simulink model "ES300A_SinVltgGenn"  (R2013b)
settings: Solver=FixedStepDiscrete  StartTime=0.0  StopTime=5  RelTol=1e-3
values from neighbouring files (symbols this model uses):
  ELECGLBPRM_PWMPERDMAX_NANOSEC_U32 = DataDict.ConfigParam    [ES300A_SinVltgGenn_DataDict.m]
  ELECGLBPRM_PWMPERDMIN_NANOSEC_U32 = DataDict.ConfigParam    [ES300A_SinVltgGenn_DataDict.m]
  SINVLTGGENN120DEG_MOTREVELEC_F32 = DataDict.Constant    [ES300A_SinVltgGenn_DataDict.m]
  SINVLTGGENN240DEG_MOTREVELEC_F32 = DataDict.Constant    [ES300A_SinVltgGenn_DataDict.m]
  SINVLTGGENN60DEG_MOTREVELEC_F32 = DataDict.Constant    [ES300A_SinVltgGenn_DataDict.m]
  SINVLTGGENNCMUOFFSTBLX_ULS_F32 = DataDict.Constant    [ES300A_SinVltgGenn_DataDict.m]
  SINVLTGGENNCMUOFFSTBLY_NANOSEC_F32 = DataDict.Constant    [ES300A_SinVltgGenn_DataDict.m]
  SinVltgGennDthrLpFilCoeff = DataDict.Calibration    [ES300A_SinVltgGenn_DataDict.m]
  SINVLTGGENNPHAONTIMAXLIM_NANOSEC_U32 = DataDict.Constant    [ES300A_SinVltgGenn_DataDict.m]
  SINVLTGGENNPHAONTISUMMAXLIM_NANOSEC_U32 = DataDict.Constant    [ES300A_SinVltgGenn_DataDict.m]
  SINVLTGGENNPHATOGNDTBL_CNT_U16 = DataDict.Constant    [ES300A_SinVltgGenn_DataDict.m]
  SINVLTGGENNPHATOGNDTBLSIZE_CNT_U16 = DataDict.Constant    [ES300A_SinVltgGenn_DataDict.m]
  SINVLTGGENNSEEDINI_ULS_F32 = DataDict.Constant    [ES300A_SinVltgGenn_DataDict.m]
  SINVLTGGENNSEEDMPLR_ULS_U08 = DataDict.Constant    [ES300A_SinVltgGenn_DataDict.m]
  SINVLTGGENNSEEDOFFS_ULS_F32 = DataDict.Constant    [ES300A_SinVltgGenn_DataDict.m]
  SINVLTGGENNZERODEG_MOTREVELEC_F32 = DataDict.Constant    [ES300A_SinVltgGenn_DataDict.m]
libraries: simulink x10, FixdToFloat x2
(part 1 of 2)
Description:
  | The High Load Stall Thermal Management algorithm protects the system from prolonged intervals of high
  | assist torque at near-stall conditions. In other words, it quickly limits large torque commands if the motor
  | velocity is below a calibratable threshold.
  |      The algorithm uses a low-pass filter (LPF) and a torque limit table to reduce the maximum allowed torque
  | command under certain operating conditions. When motor velocity is equal to or falls below the calibratable
  | threshold, the torque command is applied to the input of the low-pass filter. The output of the filter ramps up
  | and indexes into the torque limit table. The output of this table is the maximum allowed torque command. A
  | slew limit calibration governs the transition rate of the table output.
settings Model: Creator=Prerit Pramod  LastModifiedBy=wzvp6q
settings Model: ModifiedHistory=|
  | 001
  | Initial Release in new model form and new FDD structures for EA 3.0.
  | J. Kleinau
  | 13-Jun-2011
  | n/a
  | 
  | 001B
  | Revised name of input signal from PreLimitTorque to PreLimitforStall to match outputs of SF-04 Assist Sum & Limiting. Updated all references in text and on figures.
  | J. Kleinau
  | 02-Sep-2011
  | n/a
  | 
  | 002
  | Added input for serial communation service to defeat function plus definition. Cleaned up inconsistent names between sections on outputs between sections and made sure wording matched new figure names. Added Serial Comm Defeat Sub-Function section 5.5.
  | J. Kleinau
  | 08-Sep-2011
  | n/a
  | (Systems Approval and Date (N/A if not an SF FDD): Julie A. Kleinau, 08-Sep-2011; Final Approval and Date: M. Kushion, 26-Sep-2011, v002)
  | 
  | 003
  | Converted the function to a model based FDD.
  | P. Pramod
  | 09-Apr-2013
  | ICR-4051
settings DataIOCC: LimitDataPoints=off  SignalLoggingSaveFormat=ModelDataLogs  DSMLogging=off
settings OptimizationCC: ExpressionDepthLimit=2147483647
settings DebuggingCC: FcnCallInpInsideContextMsg=UseLocalSettings  StateNameClashWarn=warning
settings GRTTargetCC: CombineOutputUpdateFcns=off  GRTInterface=on

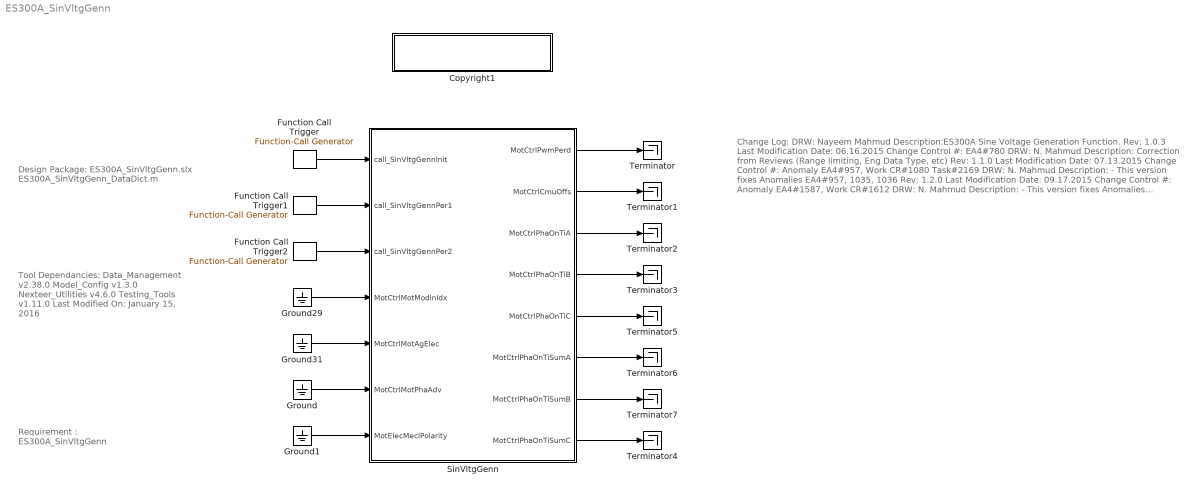
== system ES300A_SinVltgGenn ==
  note: Design Package:
      |
      | ES300A_SinVltgGenn.slx
      | ES300A_SinVltgGenn_DataDict.m
  note: Tool Dependancies:
      |
      | Data_Management v2.38.0
      | Model_Config v1.3.0
      | Nexteer_Utilities v4.6.0
      | Testing_Tools v1.11.0
      |
      | Last Modified On:
      | January 15, 2016
  note: Requirement :
      |
      | ES300A_SinVltgGenn
  note: Change Log:
      |
      | DRW: Nayeem Mahmud
      | Description:ES300A Sine Voltage Generation Function.
      |
      | Rev: 1.0.3
      | Last Modification Date: 06.16.2015
      | Change Control #: EA4#780
      | DRW: N. Mahmud
      | Description: Correction from Reviews (Range limiting, Eng Data Type, etc)
      |
      | Rev: 1.1.0
      | Last Modification Date: 07.13.2015
      | Change Control #: Anomaly EA4#957, Work CR#1080 Task#2169
      | DRW: N. Mahmud
      | Description:
      | - This version fixes  Anomalies EA4#957, 1035, 1036
      |
      | Rev: 1.2.0
      | Last Modification Date: 09.17.2015
      | Change Control #: Anomaly EA4#1587, Work CR#1612
      | DRW: N. Mahmud
      | Description:
      | - This version fixes  Anomalies EA4#1587 by removing the scaling factors for Qax, Dax
      |
      | Rev: 1.3.0
      | Last Modification Date: 01.15.2016
      | Change Control #: Anomaly EA4#1966, Work CR# EA4#3326
      | DRW: N. Mahmud
      | Description:
      | - This version fixes Anomaly EA4#1966 and clarified the requirement to
      | generate Phase On Time for the MIL testing purpose and re-establing the requirement linkage.
      | - Minor Fix: MotCtrlMotAgCorrd has been replaced by MotCtrlMotAgElec in the FR docuemnt
      |
      |
      | Rev: 1.4.0
      | Last Modification Date: 03.11.2016
      | Change Control #: Anomaly EA4#3947, Work CR# EA4#4470
      | DRW: N. Mahmud
      | Description:
      | - This version fixes Anomaly EA4#3947 for low path coverage iussue - the range of
      |  the PhaDptOffsX has been changed to -0.9999847412 to +0.9999847412 in the m-file
      |
      | Rev: 1.5.0
      | Last Modification Date: 05.06.2016
      | Change Control #: Anomaly EA4#4302, Work CR# EA4#5697
      | DRW: G.McCann
      | Description:
      | - This version fixes Anomaly EA4#4302 for .m file TestTolerance = 0 on various output signals.
      | Change to TestTolerance = 1
      | - Add datatype conversion for MotCtrlMotAgElec and MotCtrlMotPhaAdv in SinVltgGennPer1
  Copyright1 : Subsystem  Description=|  mask(Copyright Information){none=on}
      | Copyright info block.                                               
      |                                                                     
      | Place copyright information at the top of every subsystem in design.
      mask prompts: none "No parameters"
      mask help: Place copyright information at the top of every subsystem in design.
      mask Display:
      | NxtrConf = 'Nexteer Confidential';
      | 
      | sys = bdroot; %handle for the current model ("system")
      | first = get_param(sys,'Created');
      | if(isempty(first))
      |     first = datestr(now,'yyyy');
      | else
      |     first = first(end-3:end);  %year is last four digits
      | end
      | 
      | last = get_param(sys,'LastModifiedDate');
      | if isempty(last)
      |     last = datestr(now,'yyyy');
      | else
      |     last = last(end-3:end);
      | end
      | 
      | if strcmp(first,last)
      |     fprintf('%s\nCopyright  %s Nexteer',NxtrConf,first);
      | else
      |     fprintf('%s\n%s%s-%s Nexteer',NxtrConf,char(169),first,last);
      | end
  Function Call Trigger : simulink/Ports & Subsystems/Function-Call Generator  RequirementInfo={} %GIDa_42b49f65_b7bc_4fe6_8fce_d35bfefa497c  sample_time=0.000125  numberOfIterations=1
  Function Call Trigger1 : simulink/Ports & Subsystems/Function-Call Generator  RequirementInfo={} %GIDa_eccf4da5_56c7_476c_afa9_48737326cc68  sample_time=.0000625  numberOfIterations=1
  Function Call Trigger2 : simulink/Ports & Subsystems/Function-Call Generator  RequirementInfo={} %GIDa_73db9335_95f9_41b5_8685_380b234a43a2  sample_time=.0000625  numberOfIterations=1
  Ground{,1,29,31} (4 alike) : Ground
  SinVltgGenn : Subsystem
  Terminator{,1..7} (8 alike) : Terminator
  wires:
  SinVltgGenn/1(MotCtrlPwmPerd) -> Terminator/1
  SinVltgGenn/2(MotCtrlCmuOffs) -> Terminator1/1
  SinVltgGenn/3(MotCtrlPhaOnTiA) -> Terminator2/1
  SinVltgGenn/4(MotCtrlPhaOnTiB) -> Terminator3/1
  SinVltgGenn/5(MotCtrlPhaOnTiC) -> Terminator5/1
  SinVltgGenn/6(MotCtrlPhaOnTiSumA) -> Terminator6/1
  SinVltgGenn/7(MotCtrlPhaOnTiSumB) -> Terminator7/1
  SinVltgGenn/8(MotCtrlPhaOnTiSumC) -> Terminator4/1
  Function Call Trigger/1 -> SinVltgGenn/1(call_SinVltgGennInit)
  Ground1/1 -> SinVltgGenn/7(MotElecMeclPolarity)
  Ground31/1 -> SinVltgGenn/5(MotCtrlMotAgElec)
  Ground/1 -> SinVltgGenn/6(MotCtrlMotPhaAdv)
  Function Call Trigger1/1 -> SinVltgGenn/2(call_SinVltgGennPer1)
  Ground29/1 -> SinVltgGenn/4(MotCtrlMotModlnIdx)
  Function Call Trigger2/1 -> SinVltgGenn/3(call_SinVltgGennPer2)

== system ES300A_SinVltgGenn/Copyright1 ==

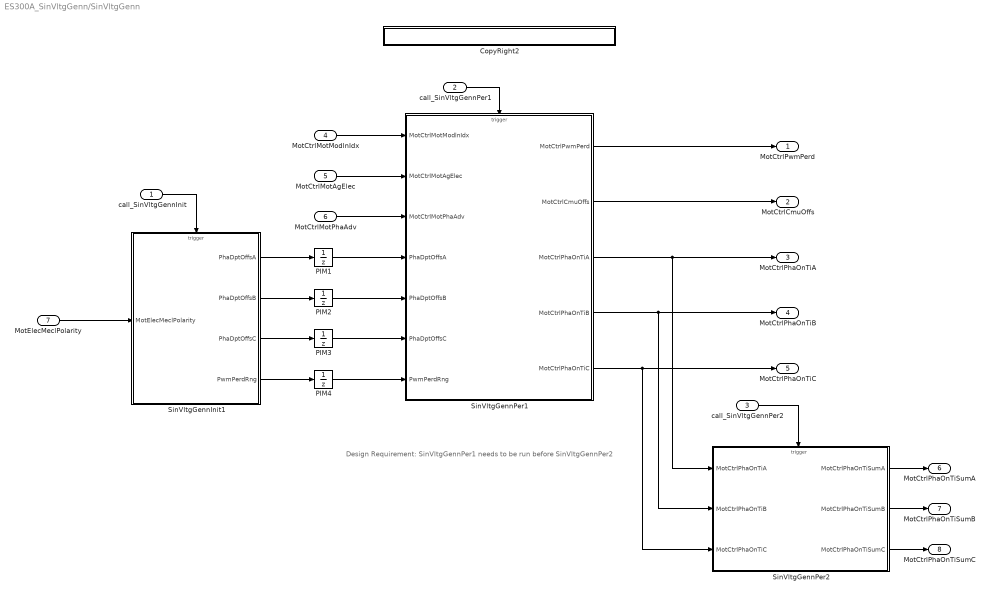
== system ES300A_SinVltgGenn/SinVltgGenn ==
  note: Design Requirement:
      |
      | SinVltgGennPer1 needs to be run before SinVltgGennPer2
  call_SinVltgGennInit : Inport
  call_SinVltgGennPer1 : Inport  RequirementInfo={'linktype_rmi_doors' '0000c478 (/ESG Group/FDD Module Requirements/EA4 Specific/ES300A_SinVltgGenn)' '#ES300A_262' 'true' 'REQ: ES300A_262' '' } %GIDa_f246c4bc_b01d_46bd_87fd_7bc120c20cb6  Port=2
  call_SinVltgGennPer2 : Inport  RequirementInfo={'linktype_rmi_doors' '0000c478 (/ESG Group/FDD Module Requirements/EA4 Specific/ES300A_SinVltgGenn)' '#ES300A_262' 'true' 'REQ: ES300A_262' '' } %GIDa_cb07c873_dffe_45e9_bd8a_092986eec373  Port=3
  MotCtrlMotModlnIdx : Inport  RequirementInfo={'linktype_rmi_doors' '0000c478 (/ESG Group/FDD Module Requirements/EA4 Specific/ES300A_SinVltgGenn)' '#ES300A_104' 'true' 'REQ: ES300A_104' '' } %GIDa_ad60892a_cd90_4ca1_a013_796fa50b9f6b  Port=4
  MotCtrlMotAgElec : Inport  RequirementInfo={'linktype_rmi_doors' '0000c478 (/ESG Group/FDD Module Requirements/EA4 Specific/ES300A_SinVltgGenn)' '#ES300A_103' 'true' 'REQ: ES300A_103' '' } %GIDa_4b3e113f_4eda_452f_adbe_4e207398b277  Port=5  OutDataTypeStr=uint16
  MotCtrlMotPhaAdv : Inport  RequirementInfo={'linktype_rmi_doors' '0000c478 (/ESG Group/FDD Module Requirements/EA4 Specific/ES300A_SinVltgGenn)' '#ES300A_102' 'true' 'REQ: ES300A_102' '' } %GIDa_539541f4_a37b_4cf3_8f66_eed52b458e12  Port=6
  MotElecMeclPolarity : Inport  RequirementInfo={'linktype_rmi_doors' '0000c478 (/ESG Group/FDD Module Requirements/EA4 Specific/ES300A_SinVltgGenn)' '#ES300A_101' 'true' 'REQ: ES300A_101' '' } %GIDa_3aacba32_bb9e_44c1_8fbe_41c187cf6531  Port=7  OutDataTypeStr=int8
  CopyRight2 : Subsystem  Description=|  mask(Copyright Information){none=on}
      | Copyright info block.                                               
      |                                                                     
      | Place copyright information at the top of every subsystem in design.
      mask prompts: none "No parameters"
      mask help: Place copyright information at the top of every subsystem in design.
      mask Display:
      | NxtrConf = 'Nexteer Confidential';
      | 
      | sys = bdroot; %handle for the current model ("system")
      | first = get_param(sys,'Created');
      | first = first(end-3:end);  %year is last four digits
      | 
      | last = get_param(sys,'LastModifiedDate');
      | if isempty(last)
      |     last = datestr(now,'yyyy');
      | else
      |     last = last(end-3:end);
      | end
      | 
      | if strcmp(first,last)
      |     fprintf('%s -- Copyright %s Nexteer',NxtrConf,first)
      | else
      |     fprintf('%s -- %s%s- %s Nexteer',NxtrConf,char(169),first,last)
      | end
  PIM1 : UnitDelay  SampleTime=-1  StateName=PhaDptOffsA  StateMustResolveToSignalObject=on
      settings: AttributesFormatString=%<StateName>
  PIM2 : UnitDelay  SampleTime=-1  StateName=PhaDptOffsB  StateMustResolveToSignalObject=on
      settings: AttributesFormatString=%<StateName>
  PIM3 : UnitDelay  SampleTime=-1  StateName=PhaDptOffsC  StateMustResolveToSignalObject=on
      settings: AttributesFormatString=%<StateName>
  PIM4 : UnitDelay  SampleTime=-1  StateName=PwmPerdRng  StateMustResolveToSignalObject=on
      settings: AttributesFormatString=%<StateName>
  SinVltgGennInit1 : Subsystem  RequirementInfo={} %GIDa_0392e040_6b5c_412d_8a7d_718d648f6278
  "SinVltgGennPer1 " : Subsystem  RequirementInfo={} %GIDa_549824ac_cd5c_4c95_a675_df6f487678c7
  SinVltgGennPer2 : Subsystem  RequirementInfo={'linktype_rmi_doors' '0000c478 (/ESG Group/FDD Module Requirements/EA4 Specific/ES300A_SinVltgGenn)' '#ES300A_222' 'true' 'REQ: ES300A_222' '' } %GIDa_76deaeb9_b1d2_459f_ad29_4b1d07dec535
  MotCtrlPwmPerd : Outport  RequirementInfo={'linktype_rmi_doors' '0000c478 (/ESG Group/FDD Module Requirements/EA4 Specific/ES300A_SinVltgGenn)' '#ES300A_205' 'true' 'REQ: ES300A_205' '' } %GIDa_6cbcbefa_aa55_4993_ad1c_4065d3fb3a3d
  MotCtrlCmuOffs : Outport  RequirementInfo={'linktype_rmi_doors' '0000c478 (/ESG Group/FDD Module Requirements/EA4 Specific/ES300A_SinVltgGenn)' '#ES300A_216' 'true' 'REQ: ES300A_216' '' } %GIDa_2b3eb6f8_9eb6_4828_96ea_6795ba24de4f  Port=2
  MotCtrlPhaOnTiA : Outport  RequirementInfo={'linktype_rmi_doors' '0000c478 (/ESG Group/FDD Module Requirements/EA4 Specific/ES300A_SinVltgGenn)' '#ES300A_268' 'true' 'REQ: ES300A_268' '' } %GIDa_ec832360_6aeb_44e8_bb3f_d0d77f82d2cb  Port=3
  MotCtrlPhaOnTiB : Outport  RequirementInfo={'linktype_rmi_doors' '0000c478 (/ESG Group/FDD Module Requirements/EA4 Specific/ES300A_SinVltgGenn)' '#ES300A_267' 'true' 'REQ: ES300A_267' '' } %GIDa_fcb902b1_b78b_434b_9714_2f5353bba401  Port=4
  MotCtrlPhaOnTiC : Outport  RequirementInfo={'linktype_rmi_doors' '0000c478 (/ESG Group/FDD Module Requirements/EA4 Specific/ES300A_SinVltgGenn)' '#ES300A_266' 'true' 'REQ: ES300A_266' '' } %GIDa_d7869026_72ad_430e_9757_795545999b2a  Port=5
  MotCtrlPhaOnTiSumA : Outport  RequirementInfo={'linktype_rmi_doors' '0000c478 (/ESG Group/FDD Module Requirements/EA4 Specific/ES300A_SinVltgGenn)' '#ES300A_265' 'true' 'REQ: ES300A_265' '' } %GIDa_48e85bf0_5576_4b4c_8922_80839e16c5af  Port=6  OutDataTypeStr=uint32
  MotCtrlPhaOnTiSumB : Outport  RequirementInfo={'linktype_rmi_doors' '0000c478 (/ESG Group/FDD Module Requirements/EA4 Specific/ES300A_SinVltgGenn)' '#ES300A_264' 'true' 'REQ: ES300A_264' '' } %GIDa_0b5f615b_9b34_4071_a723_8c24adb2ea62  Port=7  OutDataTypeStr=uint32
  MotCtrlPhaOnTiSumC : Outport  RequirementInfo={'linktype_rmi_doors' '0000c478 (/ESG Group/FDD Module Requirements/EA4 Specific/ES300A_SinVltgGenn)' '#ES300A_263' 'true' 'REQ: ES300A_263' '' } %GIDa_85a65e43_f3be_4086_8ed5_4bbe1442b3cf  Port=8  OutDataTypeStr=uint32
  wires:
  MotElecMeclPolarity/1 -> SinVltgGennInit1/1(MotElecMeclPolarity)
  SinVltgGennInit1/1(PhaDptOffsA) -> PIM1/1
  SinVltgGennInit1/2(PhaDptOffsB) -> PIM2/1
  SinVltgGennInit1/3(PhaDptOffsC) -> PIM3/1
  MotCtrlMotModlnIdx/1 -> "SinVltgGennPer1 "/1(MotCtrlMotModlnIdx)
  MotCtrlMotPhaAdv/1 -> "SinVltgGennPer1 "/3(" MotCtrlMotPhaAdv")
  MotCtrlMotAgElec/1 -> "SinVltgGennPer1 "/2("  MotCtrlMotAgElec")
  call_SinVltgGennPer1/1 -> "SinVltgGennPer1 "/Trigger
  call_SinVltgGennInit/1 -> SinVltgGennInit1/Trigger
  SinVltgGennInit1/4(PwmPerdRng) -> PIM4/1
  "SinVltgGennPer1 "/2(MotCtrlCmuOffs) -> MotCtrlCmuOffs/1
  PIM1/1 -> "SinVltgGennPer1 "/4(PhaDptOffsA)
  PIM2/1 -> "SinVltgGennPer1 "/5(PhaDptOffsB)
  PIM3/1 -> "SinVltgGennPer1 "/6(PhaDptOffsC)
  PIM4/1 -> "SinVltgGennPer1 "/7(PwmPerdRng)
  SinVltgGennPer2/1(MotCtrlPhaOnTiSumA) -> MotCtrlPhaOnTiSumA/1
  SinVltgGennPer2/2(MotCtrlPhaOnTiSumB) -> MotCtrlPhaOnTiSumB/1
  SinVltgGennPer2/3(MotCtrlPhaOnTiSumC) -> MotCtrlPhaOnTiSumC/1
  "SinVltgGennPer1 "/3(MotCtrlPhaOnTiA) -> MotCtrlPhaOnTiA/1, SinVltgGennPer2/1(MotCtrlPhaOnTiA)
  "SinVltgGennPer1 "/4(MotCtrlPhaOnTiB) -> MotCtrlPhaOnTiB/1, SinVltgGennPer2/2(MotCtrlPhaOnTiB)
  "SinVltgGennPer1 "/5(MotCtrlPhaOnTiC) -> MotCtrlPhaOnTiC/1, SinVltgGennPer2/3(MotCtrlPhaOnTiC)
  call_SinVltgGennPer2/1 -> SinVltgGennPer2/Trigger
  "SinVltgGennPer1 "/1(MotCtrlPwmPerd) -> MotCtrlPwmPerd/1

== system ES300A_SinVltgGenn/SinVltgGenn/CopyRight2 ==

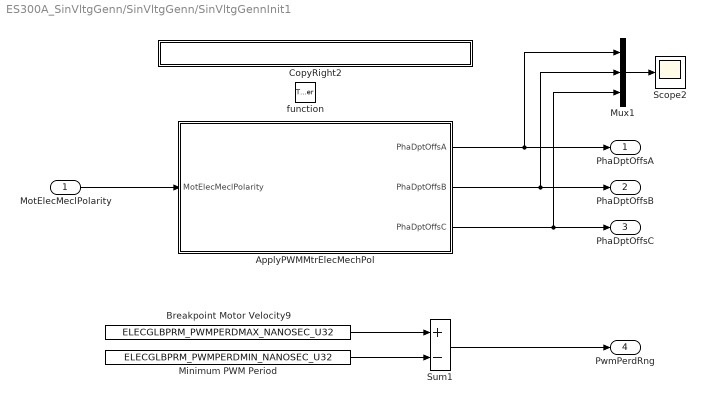
== system ES300A_SinVltgGenn/SinVltgGenn/SinVltgGennInit1 ==
  MotElecMeclPolarity : Inport
  function : TriggerPort  TriggerType=function-call
  ApplyPWMMtrElecMechPol : Subsystem  RequirementInfo={'linktype_rmi_doors' '0000c478 (/ESG Group/FDD Module Requirements/EA4 Specific/ES300A_SinVltgGenn)' '#ES300A_279' 'true' 'REQ: ES300A_279' '' ; 'linktype_rmi_doors' '0000c478 (/ESG Group/FDD Module Requirements/EA4 Specific/ES300A_SinVltgGenn)' '#ES300A_281' 'true' 'REQ: ES300A_281' '' } %GIDa_3bed5a97_331b_47d7_ae88_9b64c23aa199
  Breakpoint Motor Velocity9 : Constant  RequirementInfo={} %GIDa_5a372f5e_ce33_4aa9_8d65_800f6a5f284f  Value=ELECGLBPRM_PWMPERDMAX_NANOSEC_U32
  CopyRight2 : Subsystem  Description=|  mask(Copyright Information){none=on}
      | Copyright info block.                                               
      |                                                                     
      | Place copyright information at the top of every subsystem in design.
      mask prompts: none "No parameters"
      mask help: Place copyright information at the top of every subsystem in design.
      mask Display:
      | NxtrConf = 'Nexteer Confidential';
      | 
      | sys = bdroot; %handle for the current model ("system")
      | first = get_param(sys,'Created');
      | first = first(end-3:end);  %year is last four digits
      | 
      | last = get_param(sys,'LastModifiedDate');
      | if isempty(last)
      |     last = datestr(now,'yyyy');
      | else
      |     last = last(end-3:end);
      | end
      | 
      | if strcmp(first,last)
      |     fprintf('%s -- Copyright %s Nexteer',NxtrConf,first)
      | else
      |     fprintf('%s -- %s%s- %s Nexteer',NxtrConf,char(169),first,last)
      | end
  Minimum PWM Period : Constant  RequirementInfo={} %GIDa_584ae1b4_c7da_4213_ae12_086aa2490330  Value=ELECGLBPRM_PWMPERDMIN_NANOSEC_U32  OutDataTypeStr=uint32
  Mux1 : Mux  Inputs=3
  Scope2 : Scope
      settings: YMin=-0.35  YMax=0.35  SaveName=ScopeData9
  Sum1 : Sum  RequirementInfo={} %GIDa_fd0d5a38_a3d6_4466_bbdd_70e52ec0eded  Inputs=+-
  PhaDptOffsA : Outport  RequirementInfo={'linktype_rmi_doors' '0000c478 (/ESG Group/FDD Module Requirements/EA4 Specific/ES300A_SinVltgGenn)' '#ES300A_207' 'true' 'REQ: ES300A_207' '' ; 'linktype_rmi_doors' '0000c478 (/ESG Group/FDD Module Requirements/EA4 Specific/ES300A_SinVltgGenn)' '#ES300A_281' 'true' 'REQ: ES300A_281' '' } %GIDa_8aed702e_0aa2_4a8b_b930_0aa40450f7b1  OutDataTypeStr=single
  PhaDptOffsB : Outport  RequirementInfo={'linktype_rmi_doors' '0000c478 (/ESG Group/FDD Module Requirements/EA4 Specific/ES300A_SinVltgGenn)' '#ES300A_271' 'true' 'REQ: ES300A_271' '' ; 'linktype_rmi_doors' '0000c478 (/ESG Group/FDD Module Requirements/EA4 Specific/ES300A_SinVltgGenn)' '#ES300A_281' 'true' 'REQ: ES300A_281' '' } %GIDa_d0d9e6ef_4c07_420f_9ad6_3206178032ba  Port=2  OutDataTypeStr=single
  PhaDptOffsC : Outport  RequirementInfo={'linktype_rmi_doors' '0000c478 (/ESG Group/FDD Module Requirements/EA4 Specific/ES300A_SinVltgGenn)' '#ES300A_270' 'true' 'REQ: ES300A_270' '' ; 'linktype_rmi_doors' '0000c478 (/ESG Group/FDD Module Requirements/EA4 Specific/ES300A_SinVltgGenn)' '#ES300A_281' 'true' 'REQ: ES300A_281' '' } %GIDa_b864e084_0870_4f6e_96a6_b1cec3fbb7a1  Port=3  OutDataTypeStr=single
  PwmPerdRng : Outport  RequirementInfo={} %GIDa_196af9cb_6152_48ff_a5d5_4ccc6eece2cf  Port=4
  wires:
  ApplyPWMMtrElecMechPol/2(PhaDptOffsB) -> Mux1/2, PhaDptOffsB/1
  ApplyPWMMtrElecMechPol/3(PhaDptOffsC) -> Mux1/3, PhaDptOffsC/1
  MotElecMeclPolarity/1 -> ApplyPWMMtrElecMechPol/1(MotElecMeclPolarity)
  ApplyPWMMtrElecMechPol/1(PhaDptOffsA) -> Mux1/1, PhaDptOffsA/1
  Breakpoint Motor Velocity9/1 -> Sum1/1
  Minimum PWM Period/1 -> Sum1/2
  Mux1/1 -> Scope2/1
  Sum1/1 -> PwmPerdRng/1

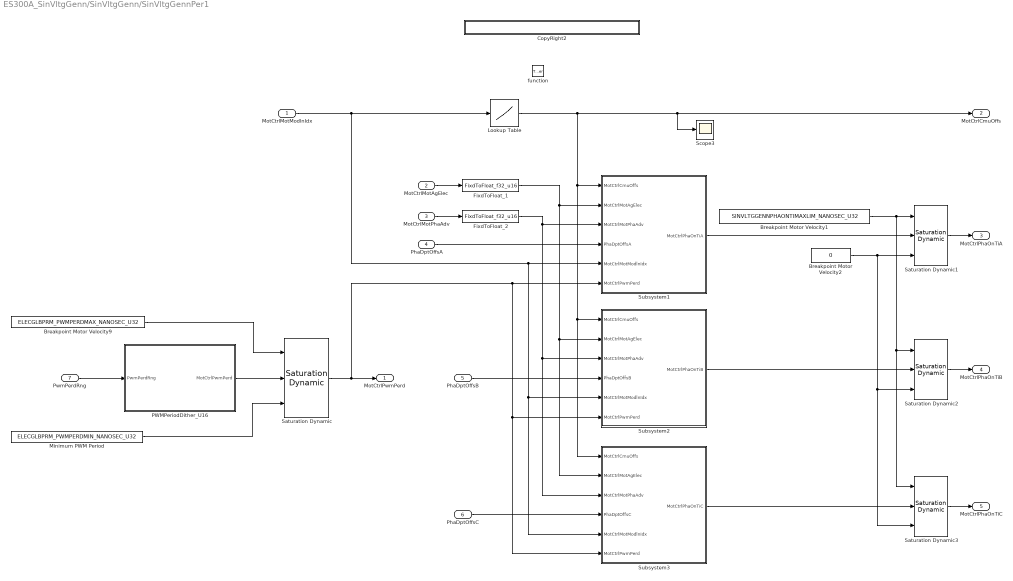
== system ES300A_SinVltgGenn/SinVltgGenn/SinVltgGennPer1  ==
  MotCtrlMotModlnIdx : Inport
  "  MotCtrlMotAgElec" : Inport  Port=2
  " MotCtrlMotPhaAdv" : Inport  Port=3
  PhaDptOffsA : Inport  Port=4
  PhaDptOffsB : Inport  Port=5
  PhaDptOffsC : Inport  Port=6
  PwmPerdRng : Inport  Port=7
  function : TriggerPort  TriggerType=function-call
  Breakpoint Motor Velocity1 : Constant  Value=SINVLTGGENNPHAONTIMAXLIM_NANOSEC_U32
  Breakpoint Motor Velocity2 : Constant  Value=0
  Breakpoint Motor Velocity9 : Constant  Value=ELECGLBPRM_PWMPERDMAX_NANOSEC_U32
  CopyRight2 : Subsystem  Description=|  mask(Copyright Information){none=on}
      | Copyright info block.                                               
      |                                                                     
      | Place copyright information at the top of every subsystem in design.
      mask prompts: none "No parameters"
      mask help: Place copyright information at the top of every subsystem in design.
      mask Display:
      | NxtrConf = 'Nexteer Confidential';
      | 
      | sys = bdroot; %handle for the current model ("system")
      | first = get_param(sys,'Created');
      | first = first(end-3:end);  %year is last four digits
      | 
      | last = get_param(sys,'LastModifiedDate');
      | if isempty(last)
      |     last = datestr(now,'yyyy');
      | else
      |     last = last(end-3:end);
      | end
      | 
      | if strcmp(first,last)
      |     fprintf('%s -- Copyright %s Nexteer',NxtrConf,first)
      | else
      |     fprintf('%s -- %s%s- %s Nexteer',NxtrConf,char(169),first,last)
      | end
  FixdToFloat_1 : FixdToFloat/FixdToFloat_f32_u16  Param1=16
      settings: AttributesFormatString=FixdToFloat_f32_u16
  FixdToFloat_2 : FixdToFloat/FixdToFloat_f32_u16  Param1=16
      settings: AttributesFormatString=FixdToFloat_f32_u16
  Lookup Table : Lookup  InputValues=SINVLTGGENNCMUOFFSTBLX_ULS_F32  Table=SINVLTGGENNCMUOFFSTBLY_NANOSEC_F32  LookUpMeth=Interpolation-Use End Values
      settings: AttributesFormatString=%<InputValues>\n%<Table>
  Minimum PWM Period : Constant  Value=ELECGLBPRM_PWMPERDMIN_NANOSEC_U32  OutDataTypeStr=uint32
  "PWMPeriodDither_U16 " : Subsystem  RequirementInfo={'linktype_rmi_doors' '0000c478 (/ESG Group/FDD Module Requirements/EA4 Specific/ES300A_SinVltgGenn)' '#ES300A_219' 'true' 'REQ: ES300A_219' '' } %GIDa_539f7f55_8bec_4b2f_b688_9ad784cb2f7b
  Saturation Dynamic : simulink/Discontinuities/Saturation Dynamic  RequirementInfo={'linktype_rmi_doors' '0000c478 (/ESG Group/FDD Module Requirements/EA4 Specific/ES300A_SinVltgGenn)' '#ES300A_278' 'true' 'REQ: ES300A_278' '' } %GIDa_dd1b5fc7_33b4_4925_9442_df73b5b51b22  OutMin=[]  OutMax=[]  OutDataTypeStr=Inherit: Same as second input  OutDataType=fixdt(1, 16)  OutScaling=2^-10  DoSatur=off
  Saturation Dynamic1 : simulink/Discontinuities/Saturation Dynamic  RequirementInfo={} %GIDa_c92aa31a_5d2a_4bbb_bcf9_69c6a9e67e9f  OutMin=[]  OutMax=[]  OutDataTypeStr=Inherit: Same as second input  OutDataType=fixdt(1, 16)  OutScaling=2^-10  DoSatur=off
  Saturation Dynamic2 : simulink/Discontinuities/Saturation Dynamic  RequirementInfo={} %GIDa_54482bc3_5ba9_4bc4_b0ff_db35c96ac17d  OutMin=[]  OutMax=[]  OutDataTypeStr=Inherit: Same as second input  OutDataType=fixdt(1, 16)  OutScaling=2^-10  DoSatur=off
  Saturation Dynamic3 : simulink/Discontinuities/Saturation Dynamic  RequirementInfo={} %GIDa_582ab7c2_51f7_472a_af65_d82acec897a3  OutMin=[]  OutMax=[]  OutDataTypeStr=Inherit: Same as second input  OutDataType=fixdt(1, 16)  OutScaling=2^-10  DoSatur=off
  Scope3 : Scope
      settings: YMin=3125  YMax=3125
  Subsystem1 : Subsystem  RequirementInfo={'linktype_rmi_doors' '0000c478 (/ESG Group/FDD Module Requirements/EA4 Specific/ES300A_SinVltgGenn)' '#ES300A_211' 'true' 'REQ: ES300A_211' '' ; 'linktype_rmi_doors' '0000c478 (/ESG Group/FDD Module Requirements/EA4 Specific/ES300A_SinVltgGenn)' '#ES300A_211' 'true' 'REQ: ES300A_211' '' ; 'linktype_rmi_doors' '0000c478 (/ESG Group/FDD Module Requirements/EA4 Specific/ES300A_SinVltgGenn)' '#ES300A_283' 'true' 'REQ: ES300A_283' '' ; 'linktype_rmi_doors' '0000c478 (/ESG Group/FDD Module Requirements/EA4 Specific/ES300A_SinVltgGenn)' '#ES300A_282' 'true' 'REQ: ES300A_282' '' } %GIDa_b60b92ec_8908_41c8_b4ba_c1a85855e6b6
  Subsystem2 : Subsystem  RequirementInfo={'linktype_rmi_doors' '0000c478 (/ESG Group/FDD Module Requirements/EA4 Specific/ES300A_SinVltgGenn)' '#ES300A_211' 'true' 'REQ: ES300A_211' '' ; 'linktype_rmi_doors' '0000c478 (/ESG Group/FDD Module Requirements/EA4 Specific/ES300A_SinVltgGenn)' '#ES300A_211' 'true' 'REQ: ES300A_211' '' ; 'linktype_rmi_doors' '0000c478 (/ESG Group/FDD Module Requirements/EA4 Specific/ES300A_SinVltgGenn)' '#ES300A_283' 'true' 'REQ: ES300A_283' '' ; 'linktype_rmi_doors' '0000c478 (/ESG Group/FDD Module Requirements/EA4 Specific/ES300A_SinVltgGenn)' '#ES300A_282' 'true' 'REQ: ES300A_282' '' } %GIDa_9c59f437_716a_4eaa_a19a_f7cf56a49256
  Subsystem3 : Subsystem  RequirementInfo={'linktype_rmi_doors' '0000c478 (/ESG Group/FDD Module Requirements/EA4 Specific/ES300A_SinVltgGenn)' '#ES300A_211' 'true' 'REQ: ES300A_211' '' ; 'linktype_rmi_doors' '0000c478 (/ESG Group/FDD Module Requirements/EA4 Specific/ES300A_SinVltgGenn)' '#ES300A_211' 'true' 'REQ: ES300A_211' '' ; 'linktype_rmi_doors' '0000c478 (/ESG Group/FDD Module Requirements/EA4 Specific/ES300A_SinVltgGenn)' '#ES300A_283' 'true' 'REQ: ES300A_283' '' ; 'linktype_rmi_doors' '0000c478 (/ESG Group/FDD Module Requirements/EA4 Specific/ES300A_SinVltgGenn)' '#ES300A_282' 'true' 'REQ: ES300A_282' '' } %GIDa_9bcce658_297c_4fd2_a0fc_4ec3498cd570
  MotCtrlPwmPerd : Outport  RequirementInfo={'linktype_rmi_doors' '0000c478 (/ESG Group/FDD Module Requirements/EA4 Specific/ES300A_SinVltgGenn)' '#ES300A_15' 'true' 'REQ: ES300A_15' '' } %GIDa_45ef2ca4_5d39_497e_8f89_cad989cd8515  OutDataTypeStr=uint32
  MotCtrlCmuOffs : Outport  Port=2
  MotCtrlPhaOnTiA : Outport  RequirementInfo={'linktype_rmi_doors' '0000c478 (/ESG Group/FDD Module Requirements/EA4 Specific/ES300A_SinVltgGenn)' '#ES300A_277' 'true' 'REQ: ES300A_277' '' } %GIDa_4a167b8d_0395_4a15_a252_1fdb2642f3bb  Port=3  OutDataTypeStr=uint32
  MotCtrlPhaOnTiB : Outport  RequirementInfo={'linktype_rmi_doors' '0000c478 (/ESG Group/FDD Module Requirements/EA4 Specific/ES300A_SinVltgGenn)' '#ES300A_277' 'true' 'REQ: ES300A_277' '' } %GIDa_908261c8_1d22_4358_92cf_915e8b18fba9  Port=4  OutDataTypeStr=uint32
  MotCtrlPhaOnTiC : Outport  RequirementInfo={'linktype_rmi_doors' '0000c478 (/ESG Group/FDD Module Requirements/EA4 Specific/ES300A_SinVltgGenn)' '#ES300A_277' 'true' 'REQ: ES300A_277' '' } %GIDa_30bc8a1b_5332_4fac_b802_5011b9defb9f  Port=5  OutDataTypeStr=uint32
  wires:
  Subsystem1/1(MotCtrlPhaOnTiA) -> Saturation Dynamic1/2
  Minimum PWM Period/1 -> Saturation Dynamic/3
  Breakpoint Motor Velocity9/1 -> Saturation Dynamic/1
  Saturation Dynamic/1 -> Subsystem1/6(MotCtrlPwmPerd), Subsystem2/6(MotCtrlPwmPerd), Subsystem3/6(MotCtrlPwmPerd), MotCtrlPwmPerd/1
  "  MotCtrlMotAgElec"/1 -> FixdToFloat_1/1
  "PWMPeriodDither_U16 "/1(MotCtrlPwmPerd) -> Saturation Dynamic/2
  " MotCtrlMotPhaAdv"/1 -> FixdToFloat_2/1
  PhaDptOffsA/1 -> Subsystem1/4(PhaDptOffsA)
  MotCtrlMotModlnIdx/1 -> Lookup Table/1, Subsystem1/5(MotCtrlMotModlnIdx), Subsystem2/5(MotCtrlMotModlnIdx), Subsystem3/5(MotCtrlMotModlnIdx)
  PwmPerdRng/1 -> "PWMPeriodDither_U16 "/1(PwmPerdRng)
  Lookup Table/1 -> Scope3/1, MotCtrlCmuOffs/1, Subsystem3/1(MotCtrlCmuOffs), Subsystem2/1(MotCtrlCmuOffs), Subsystem1/1(MotCtrlCmuOffs)
  PhaDptOffsB/1 -> Subsystem2/4(PhaDptOffsB)
  PhaDptOffsC/1 -> Subsystem3/4(PhaDptOffsC)
  Saturation Dynamic1/1 -> MotCtrlPhaOnTiA/1
  Subsystem2/1(MotCtrlPhaOnTiB) -> Saturation Dynamic2/2
  Saturation Dynamic2/1 -> MotCtrlPhaOnTiB/1
  Subsystem3/1(MotCtrlPhaOnTiC) -> Saturation Dynamic3/2
  Saturation Dynamic3/1 -> MotCtrlPhaOnTiC/1
  Breakpoint Motor Velocity1/1 -> Saturation Dynamic2/1, Saturation Dynamic3/1, Saturation Dynamic1/1
  Breakpoint Motor Velocity2/1 -> Saturation Dynamic2/3, Saturation Dynamic3/3, Saturation Dynamic1/3
  FixdToFloat_1/1 -> Subsystem1/2(MotCtrlMotAgElec), Subsystem2/2(MotCtrlMotAgElec), Subsystem3/2(MotCtrlMotAgElec)
  FixdToFloat_2/1 -> Subsystem2/3(MotCtrlMotPhaAdv), Subsystem3/3(MotCtrlMotPhaAdv), Subsystem1/3(MotCtrlMotPhaAdv)

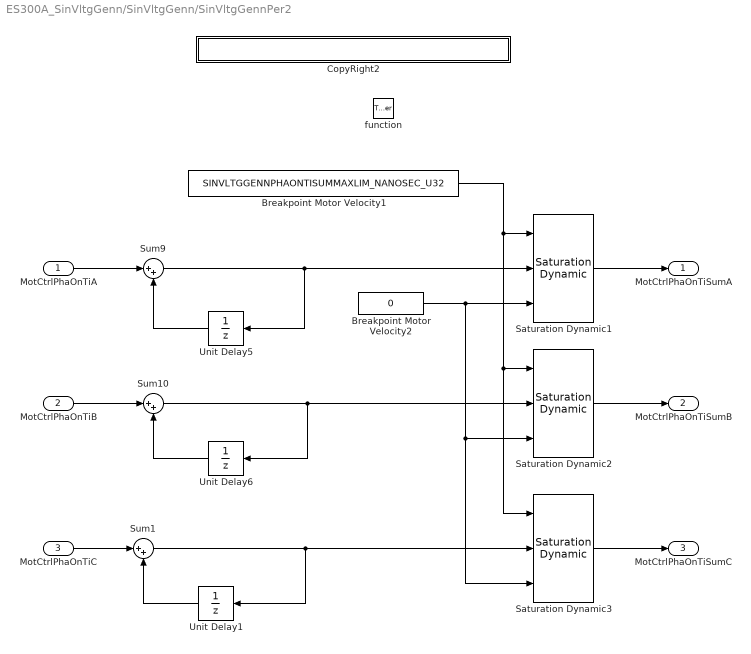
== system ES300A_SinVltgGenn/SinVltgGenn/SinVltgGennPer2 ==
  MotCtrlPhaOnTiA : Inport  OutDataTypeStr=uint32
  MotCtrlPhaOnTiB : Inport  Port=2
  MotCtrlPhaOnTiC : Inport  Port=3
  function : TriggerPort  TriggerType=function-call
  Breakpoint Motor Velocity1 : Constant  Value=SINVLTGGENNPHAONTISUMMAXLIM_NANOSEC_U32
  Breakpoint Motor Velocity2 : Constant  Value=0
  CopyRight2 : Subsystem  Description=|  mask(Copyright Information){none=on}
      | Copyright info block.                                               
      |                                                                     
      | Place copyright information at the top of every subsystem in design.
      mask prompts: none "No parameters"
      mask help: Place copyright information at the top of every subsystem in design.
      mask Display:
      | NxtrConf = 'Nexteer Confidential';
      | 
      | sys = bdroot; %handle for the current model ("system")
      | first = get_param(sys,'Created');
      | first = first(end-3:end);  %year is last four digits
      | 
      | last = get_param(sys,'LastModifiedDate');
      | if isempty(last)
      |     last = datestr(now,'yyyy');
      | else
      |     last = last(end-3:end);
      | end
      | 
      | if strcmp(first,last)
      |     fprintf('%s -- Copyright %s Nexteer',NxtrConf,first)
      | else
      |     fprintf('%s -- %s%s- %s Nexteer',NxtrConf,char(169),first,last)
      | end
  Saturation Dynamic1 : simulink/Discontinuities/Saturation Dynamic  RequirementInfo={} %GIDa_b2e439e8_2b96_4728_989a_5160d6be1599  OutMin=[]  OutMax=[]  OutDataTypeStr=Inherit: Same as second input  OutDataType=fixdt(1, 16)  OutScaling=2^-10  DoSatur=off
  Saturation Dynamic2 : simulink/Discontinuities/Saturation Dynamic  RequirementInfo={} %GIDa_eba5d9c8_8d09_49e6_ad75_2da52f228460  OutMin=[]  OutMax=[]  OutDataTypeStr=Inherit: Same as second input  OutDataType=fixdt(1, 16)  OutScaling=2^-10  DoSatur=off
  Saturation Dynamic3 : simulink/Discontinuities/Saturation Dynamic  RequirementInfo={} %GIDa_90f2fdc0_48a3_420d_a4ef_dfe7f19658fc  OutMin=[]  OutMax=[]  OutDataTypeStr=Inherit: Same as second input  OutDataType=fixdt(1, 16)  OutScaling=2^-10  DoSatur=off
  Sum1 : Sum  Inputs=|++  AccumDataTypeStr=uint32
  Sum10 : Sum  Inputs=|++  AccumDataTypeStr=uint32
  Sum9 : Sum  Inputs=|++  AccumDataTypeStr=uint32
  Unit Delay1 : UnitDelay  SampleTime=-1  StateName=PhaOnTiSumCPrev  StateMustResolveToSignalObject=on
      settings: AttributesFormatString=%<StateName>
  Unit Delay5 : UnitDelay  SampleTime=-1  StateName=PhaOnTiSumAPrev  StateMustResolveToSignalObject=on
      settings: AttributesFormatString=%<StateName>
  Unit Delay6 : UnitDelay  SampleTime=-1  StateName=PhaOnTiSumBPrev  StateMustResolveToSignalObject=on
      settings: AttributesFormatString=%<StateName>
  MotCtrlPhaOnTiSumA : Outport  RequirementInfo={'linktype_rmi_doors' '0000c478 (/ESG Group/FDD Module Requirements/EA4 Specific/ES300A_SinVltgGenn)' '#ES300A_276' 'true' 'REQ: ES300A_276' '' } %GIDa_a5db1705_0f34_45dd_ab42_0e8faf5ec1c6  OutDataTypeStr=uint32
  MotCtrlPhaOnTiSumB : Outport  RequirementInfo={'linktype_rmi_doors' '0000c478 (/ESG Group/FDD Module Requirements/EA4 Specific/ES300A_SinVltgGenn)' '#ES300A_276' 'true' 'REQ: ES300A_276' '' } %GIDa_0722fe0d_1eba_4ee1_9ebf_146e6c7ad0aa  Port=2  OutDataTypeStr=uint32
  MotCtrlPhaOnTiSumC : Outport  RequirementInfo={'linktype_rmi_doors' '0000c478 (/ESG Group/FDD Module Requirements/EA4 Specific/ES300A_SinVltgGenn)' '#ES300A_276' 'true' 'REQ: ES300A_276' '' } %GIDa_c217a1e9_4013_4ffd_ad4d_dc3a9996a73b  Port=3  OutDataTypeStr=uint32
  wires:
  Sum9/1 -> Saturation Dynamic1/2, Unit Delay5/1
  Unit Delay5/1 -> Sum9/2
  Unit Delay6/1 -> Sum10/2
  Sum10/1 -> Saturation Dynamic2/2, Unit Delay6/1
  MotCtrlPhaOnTiA/1 -> Sum9/1
  MotCtrlPhaOnTiB/1 -> Sum10/1
  Unit Delay1/1 -> Sum1/2
  Sum1/1 -> Saturation Dynamic3/2, Unit Delay1/1
  MotCtrlPhaOnTiC/1 -> Sum1/1
  Saturation Dynamic1/1 -> MotCtrlPhaOnTiSumA/1
  Saturation Dynamic2/1 -> MotCtrlPhaOnTiSumB/1
  Saturation Dynamic3/1 -> MotCtrlPhaOnTiSumC/1
  Breakpoint Motor Velocity1/1 -> Saturation Dynamic3/1, Saturation Dynamic2/1, Saturation Dynamic1/1
  Breakpoint Motor Velocity2/1 -> Saturation Dynamic3/3, Saturation Dynamic2/3, Saturation Dynamic1/3

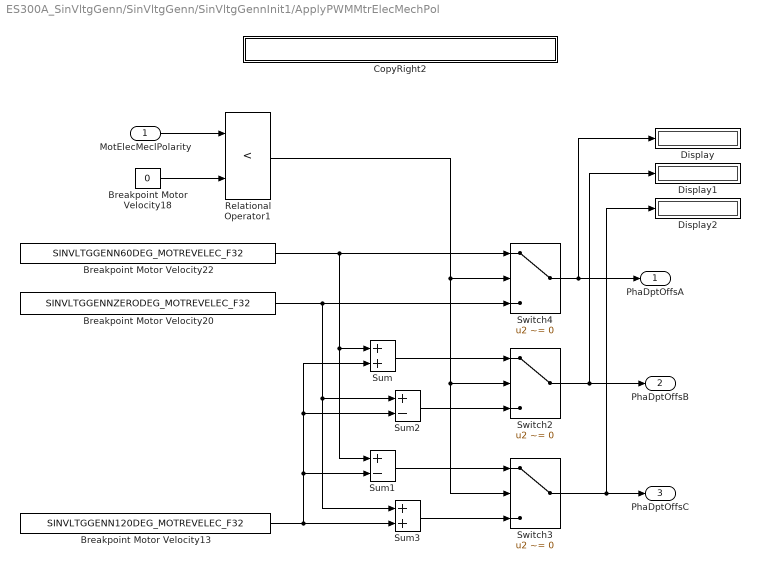
== system ES300A_SinVltgGenn/SinVltgGenn/SinVltgGennInit1/ApplyPWMMtrElecMechPol ==
  MotElecMeclPolarity : Inport
  Breakpoint Motor Velocity13 : Constant  Value=SINVLTGGENN120DEG_MOTREVELEC_F32
  Breakpoint Motor Velocity18 : Constant  Value=0
  Breakpoint Motor Velocity20 : Constant  Value=SINVLTGGENNZERODEG_MOTREVELEC_F32
  Breakpoint Motor Velocity22 : Constant  Value=SINVLTGGENN60DEG_MOTREVELEC_F32
  CopyRight2 : Subsystem  Description=|  mask(Copyright Information){none=on}
      | Copyright info block.                                               
      |                                                                     
      | Place copyright information at the top of every subsystem in design.
      mask prompts: none "No parameters"
      mask help: Place copyright information at the top of every subsystem in design.
      mask Display:
      | NxtrConf = 'Nexteer Confidential';
      | 
      | sys = bdroot; %handle for the current model ("system")
      | first = get_param(sys,'Created');
      | first = first(end-3:end);  %year is last four digits
      | 
      | last = get_param(sys,'LastModifiedDate');
      | if isempty(last)
      |     last = datestr(now,'yyyy');
      | else
      |     last = last(end-3:end);
      | end
      | 
      | if strcmp(first,last)
      |     fprintf('%s -- Copyright %s Nexteer',NxtrConf,first)
      | else
      |     fprintf('%s -- %s%s- %s Nexteer',NxtrConf,char(169),first,last)
      | end
  Display : Display
  Display1 : Display
  Display2 : Display
  Relational Operator1 : RelationalOperator  Operator=<  OutDataTypeStr=boolean
  Sum : Sum
  Sum1 : Sum  Inputs=+-
  Sum2 : Sum  Inputs=+-
  Sum3 : Sum
  Switch2 : Switch  Criteria=u2 ~= 0
  Switch3 : Switch  Criteria=u2 ~= 0
  Switch4 : Switch  Criteria=u2 ~= 0
  PhaDptOffsA : Outport
  PhaDptOffsB : Outport  Port=2
  PhaDptOffsC : Outport  Port=3
  wires:
  Sum1/1 -> Switch3/1
  Sum/1 -> Switch2/1
  Sum2/1 -> Switch2/3
  Sum3/1 -> Switch3/3
  Relational Operator1/1 -> Switch3/2, Switch2/2, Switch4/2
  Switch4/1 -> Display/1, PhaDptOffsA/1
  Switch2/1 -> Display1/1, PhaDptOffsB/1
  MotElecMeclPolarity/1 -> Relational Operator1/1
  Breakpoint Motor Velocity18/1 -> Relational Operator1/2
  Breakpoint Motor Velocity13/1 -> Sum/2, Sum2/2, Sum1/2, Sum3/2
  Switch3/1 -> Display2/1, PhaDptOffsC/1
  Breakpoint Motor Velocity20/1 -> Sum2/1, Sum3/1, Switch4/3
  Breakpoint Motor Velocity22/1 -> Sum1/1, Sum/1, Switch4/1

== system ES300A_SinVltgGenn/SinVltgGenn/SinVltgGennInit1/CopyRight2 ==

== system ES300A_SinVltgGenn/SinVltgGenn/SinVltgGennPer1 /CopyRight2 ==

== system ES300A_SinVltgGenn/SinVltgGenn/SinVltgGennPer1 /PWMPeriodDither_U16  ==
  note: Simulation Purppose Only
  PwmPerdRng : Inport
  Breakpoint Motor Velocity1 : Constant  RequirementInfo={} %GIDa_1e4eb606_999c_494a_bd0c_747d2cad1b6f  Value=0  OutDataTypeStr=uint32
  Breakpoint Motor Velocity9 : Constant  RequirementInfo={} %GIDa_1eca751c_3bc7_45cc_bb4c_1b755b0002be  Value=ELECGLBPRM_PWMPERDMIN_NANOSEC_U32
  CopyRight2 : Subsystem  Description=|  mask(Copyright Information){none=on}
      | Copyright info block.                                               
      |                                                                     
      | Place copyright information at the top of every subsystem in design.
      mask prompts: none "No parameters"
      mask help: Place copyright information at the top of every subsystem in design.
      mask Display:
      | NxtrConf = 'Nexteer Confidential';
      | 
      | sys = bdroot; %handle for the current model ("system")
      | first = get_param(sys,'Created');
      | first = first(end-3:end);  %year is last four digits
      | 
      | last = get_param(sys,'LastModifiedDate');
      | if isempty(last)
      |     last = datestr(now,'yyyy');
      | else
      |     last = last(end-3:end);
      | end
      | 
      | if strcmp(first,last)
      |     fprintf('%s -- Copyright %s Nexteer',NxtrConf,first)
      | else
      |     fprintf('%s -- %s%s- %s Nexteer',NxtrConf,char(169),first,last)
      | end
  Data Type Conversion1 : DataTypeConversion  OutDataTypeStr=uint32
  Dither On/Off : ManualSwitch  CurrentSetting=0
  Filter1 : Subsystem
  Filter2 : Subsystem
  Product1 : Product  RndMeth=Zero
  RandomNumberGenerator : Subsystem
  Sum5 : Sum  Inputs=|++
  MotCtrlPwmPerd : Outport
  wires:
  Breakpoint Motor Velocity9/1 -> Sum5/2
  Product1/1 -> Filter1/1(RawPWMDither)
  Filter2/1(PwmPerdDither) -> Data Type Conversion1/1
  RandomNumberGenerator/1(RndNr) -> Product1/2
  Filter1/1(PWMPeriodFilt2Inp) -> Filter2/1(PWMPeriodFilt2Inp)
  Sum5/1 -> MotCtrlPwmPerd/1
  Data Type Conversion1/1 -> Dither On/Off/2
  PwmPerdRng/1 -> Product1/1
  Dither On/Off/1 -> Sum5/1
  Breakpoint Motor Velocity1/1 -> Dither On/Off/1

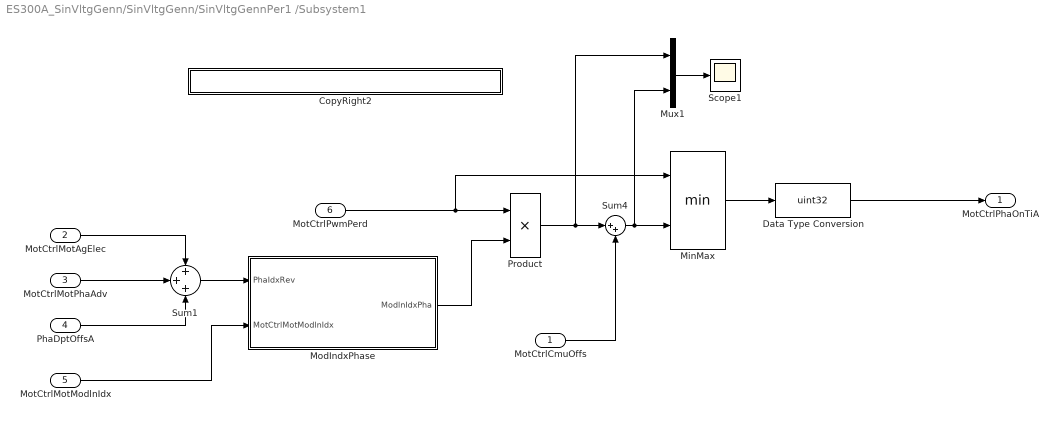
== system ES300A_SinVltgGenn/SinVltgGenn/SinVltgGennPer1 /Subsystem1 ==
  MotCtrlCmuOffs : Inport
  MotCtrlMotAgElec : Inport  Port=2
  MotCtrlMotPhaAdv : Inport  Port=3
  PhaDptOffsA : Inport  Port=4
  MotCtrlMotModlnIdx : Inport  Port=5
  MotCtrlPwmPerd : Inport  Port=6
  CopyRight2 : Subsystem  Description=|  mask(Copyright Information){none=on}
      | Copyright info block.                                               
      |                                                                     
      | Place copyright information at the top of every subsystem in design.
      mask prompts: none "No parameters"
      mask help: Place copyright information at the top of every subsystem in design.
      mask Display:
      | NxtrConf = 'Nexteer Confidential';
      | 
      | sys = bdroot; %handle for the current model ("system")
      | first = get_param(sys,'Created');
      | first = first(end-3:end);  %year is last four digits
      | 
      | last = get_param(sys,'LastModifiedDate');
      | if isempty(last)
      |     last = datestr(now,'yyyy');
      | else
      |     last = last(end-3:end);
      | end
      | 
      | if strcmp(first,last)
      |     fprintf('%s -- Copyright %s Nexteer',NxtrConf,first)
      | else
      |     fprintf('%s -- %s%s- %s Nexteer',NxtrConf,char(169),first,last)
      | end
  Data Type Conversion : DataTypeConversion  OutDataTypeStr=uint32
  MinMax : MinMax  Inputs=2
  ModIndxPhase : Subsystem
  Mux1 : Mux  Inputs=2
  Product : Product
  Scope1 : Scope
      settings: YMin=26000  YMax=39000  SaveName=ScopeData8
  Sum1 : Sum  Inputs=+++
  Sum4 : Sum  Inputs=|++
  MotCtrlPhaOnTiA : Outport  OutDataTypeStr=uint32
  wires:
  MinMax/1 -> Data Type Conversion/1
  Sum4/1 -> Mux1/2, MinMax/2
  Sum1/1 -> ModIndxPhase/1("PhaIdxRev ")
  Product/1 -> Mux1/1, Sum4/1
  ModIndxPhase/1(ModlnIdxPha) -> Product/2
  MotCtrlPwmPerd/1 -> MinMax/1, Product/1
  MotCtrlMotModlnIdx/1 -> ModIndxPhase/2(MotCtrlMotModlnIdx)
  MotCtrlMotAgElec/1 -> Sum1/1
  MotCtrlMotPhaAdv/1 -> Sum1/2
  PhaDptOffsA/1 -> Sum1/3
  Data Type Conversion/1 -> MotCtrlPhaOnTiA/1
  Mux1/1 -> Scope1/1
  MotCtrlCmuOffs/1 -> Sum4/2

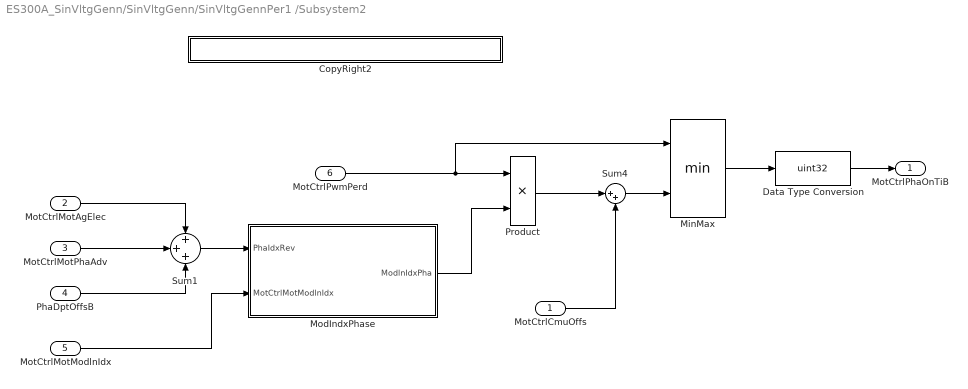
== system ES300A_SinVltgGenn/SinVltgGenn/SinVltgGennPer1 /Subsystem2 ==
  MotCtrlCmuOffs : Inport
  MotCtrlMotAgElec : Inport  Port=2
  MotCtrlMotPhaAdv : Inport  Port=3
  PhaDptOffsB : Inport  Port=4
  MotCtrlMotModlnIdx : Inport  Port=5
  MotCtrlPwmPerd : Inport  Port=6
  CopyRight2 : Subsystem  Description=|  mask(Copyright Information){none=on}
      | Copyright info block.                                               
      |                                                                     
      | Place copyright information at the top of every subsystem in design.
      mask prompts: none "No parameters"
      mask help: Place copyright information at the top of every subsystem in design.
      mask Display:
      | NxtrConf = 'Nexteer Confidential';
      | 
      | sys = bdroot; %handle for the current model ("system")
      | first = get_param(sys,'Created');
      | first = first(end-3:end);  %year is last four digits
      | 
      | last = get_param(sys,'LastModifiedDate');
      | if isempty(last)
      |     last = datestr(now,'yyyy');
      | else
      |     last = last(end-3:end);
      | end
      | 
      | if strcmp(first,last)
      |     fprintf('%s -- Copyright %s Nexteer',NxtrConf,first)
      | else
      |     fprintf('%s -- %s%s- %s Nexteer',NxtrConf,char(169),first,last)
      | end
  Data Type Conversion : DataTypeConversion  OutDataTypeStr=uint32
  MinMax : MinMax  Inputs=2
  ModIndxPhase : Subsystem
  Product : Product
  Sum1 : Sum  Inputs=+++
  Sum4 : Sum  Inputs=|++
  MotCtrlPhaOnTiB : Outport  OutDataTypeStr=uint32
  wires:
  MinMax/1 -> Data Type Conversion/1
  Sum4/1 -> MinMax/2
  Sum1/1 -> ModIndxPhase/1("PhaIdxRev ")
  MotCtrlCmuOffs/1 -> Sum4/2
  Product/1 -> Sum4/1
  ModIndxPhase/1(ModlnIdxPha) -> Product/2
  MotCtrlPwmPerd/1 -> MinMax/1, Product/1
  MotCtrlMotModlnIdx/1 -> ModIndxPhase/2(MotCtrlMotModlnIdx)
  MotCtrlMotAgElec/1 -> Sum1/1
  MotCtrlMotPhaAdv/1 -> Sum1/2
  PhaDptOffsB/1 -> Sum1/3
  Data Type Conversion/1 -> MotCtrlPhaOnTiB/1

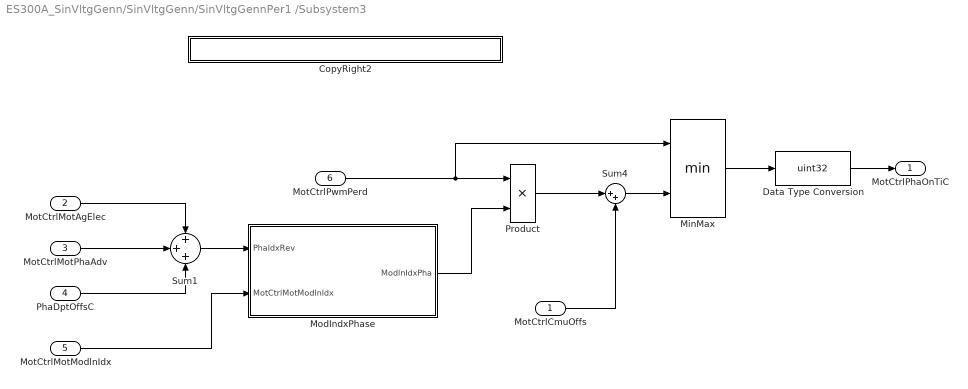
== system ES300A_SinVltgGenn/SinVltgGenn/SinVltgGennPer1 /Subsystem3 ==
  MotCtrlCmuOffs : Inport
  MotCtrlMotAgElec : Inport  Port=2
  MotCtrlMotPhaAdv : Inport  Port=3
  PhaDptOffsC : Inport  Port=4
  MotCtrlMotModlnIdx : Inport  Port=5
  MotCtrlPwmPerd : Inport  Port=6
  CopyRight2 : Subsystem  Description=|  mask(Copyright Information){none=on}
      | Copyright info block.                                               
      |                                                                     
      | Place copyright information at the top of every subsystem in design.
      mask prompts: none "No parameters"
      mask help: Place copyright information at the top of every subsystem in design.
      mask Display:
      | NxtrConf = 'Nexteer Confidential';
      | 
      | sys = bdroot; %handle for the current model ("system")
      | first = get_param(sys,'Created');
      | first = first(end-3:end);  %year is last four digits
      | 
      | last = get_param(sys,'LastModifiedDate');
      | if isempty(last)
      |     last = datestr(now,'yyyy');
      | else
      |     last = last(end-3:end);
      | end
      | 
      | if strcmp(first,last)
      |     fprintf('%s -- Copyright %s Nexteer',NxtrConf,first)
      | else
      |     fprintf('%s -- %s%s- %s Nexteer',NxtrConf,char(169),first,last)
      | end
  Data Type Conversion : DataTypeConversion  OutDataTypeStr=uint32
  MinMax : MinMax  Inputs=2
  ModIndxPhase : Subsystem
  Product : Product
  Sum1 : Sum  Inputs=+++
  Sum4 : Sum  Inputs=|++
  MotCtrlPhaOnTiC : Outport  OutDataTypeStr=uint32
  wires:
  MinMax/1 -> Data Type Conversion/1
  Sum4/1 -> MinMax/2
  Sum1/1 -> ModIndxPhase/1("PhaIdxRev ")
  MotCtrlCmuOffs/1 -> Sum4/2
  Product/1 -> Sum4/1
  ModIndxPhase/1(ModlnIdxPha) -> Product/2
  MotCtrlPwmPerd/1 -> MinMax/1, Product/1
  MotCtrlMotModlnIdx/1 -> ModIndxPhase/2(MotCtrlMotModlnIdx)
  MotCtrlMotAgElec/1 -> Sum1/1
  MotCtrlMotPhaAdv/1 -> Sum1/2
  PhaDptOffsC/1 -> Sum1/3
  Data Type Conversion/1 -> MotCtrlPhaOnTiC/1

== system ES300A_SinVltgGenn/SinVltgGenn/SinVltgGennPer2/CopyRight2 ==

== system ES300A_SinVltgGenn/SinVltgGenn/SinVltgGennInit1/ApplyPWMMtrElecMechPol/CopyRight2 ==

== system ES300A_SinVltgGenn/SinVltgGenn/SinVltgGennPer1 /PWMPeriodDither_U16 /CopyRight2 ==

== system ES300A_SinVltgGenn/SinVltgGenn/SinVltgGennPer1 /PWMPeriodDither_U16 /Filter1 ==
  RawPWMDither : Inport
  Breakpoint Motor Velocity1 : Constant  Value=SinVltgGennDthrLpFilCoeff
  CopyRight2 : Subsystem  Description=|  mask(Copyright Information){none=on}
      | Copyright info block.                                               
      |                                                                     
      | Place copyright information at the top of every subsystem in design.
      mask prompts: none "No parameters"
      mask help: Place copyright information at the top of every subsystem in design.
      mask Display:
      | NxtrConf = 'Nexteer Confidential';
      | 
      | sys = bdroot; %handle for the current model ("system")
      | first = get_param(sys,'Created');
      | first = first(end-3:end);  %year is last four digits
      | 
      | last = get_param(sys,'LastModifiedDate');
      | if isempty(last)
      |     last = datestr(now,'yyyy');
      | else
      |     last = last(end-3:end);
      | end
      | 
      | if strcmp(first,last)
      |     fprintf('%s -- Copyright %s Nexteer',NxtrConf,first)
      | else
      |     fprintf('%s -- %s%s- %s Nexteer',NxtrConf,char(169),first,last)
      | end
  Product2 : Product  RndMeth=Zero
  Scope1 : Scope
      settings: SaveName=ScopeData3
  Sum1 : Sum  Inputs=|++
  Sum3 : Sum  Inputs=|+-
  Unit Delay : UnitDelay  SampleTime=-1  StateName=Fil1OutpPrev  StateMustResolveToSignalObject=on
      settings: AttributesFormatString=%<StateName>
  PWMPeriodFilt2Inp : Outport
  wires:
  Unit Delay/1 -> Sum1/2, Sum3/2
  RawPWMDither/1 -> Sum3/1
  Sum3/1 -> Product2/2
  Product2/1 -> Sum1/1
  Breakpoint Motor Velocity1/1 -> Product2/1
  Sum1/1 -> Scope1/1, PWMPeriodFilt2Inp/1, Unit Delay/1

== system ES300A_SinVltgGenn/SinVltgGenn/SinVltgGennPer1 /PWMPeriodDither_U16 /Filter2 ==
  PWMPeriodFilt2Inp : Inport
  Breakpoint Motor Velocity3 : Constant  Value=SinVltgGennDthrLpFilCoeff
  CopyRight2 : Subsystem  Description=|  mask(Copyright Information){none=on}
      | Copyright info block.                                               
      |                                                                     
      | Place copyright information at the top of every subsystem in design.
      mask prompts: none "No parameters"
      mask help: Place copyright information at the top of every subsystem in design.
      mask Display:
      | NxtrConf = 'Nexteer Confidential';
      | 
      | sys = bdroot; %handle for the current model ("system")
      | first = get_param(sys,'Created');
      | first = first(end-3:end);  %year is last four digits
      | 
      | last = get_param(sys,'LastModifiedDate');
      | if isempty(last)
      |     last = datestr(now,'yyyy');
      | else
      |     last = last(end-3:end);
      | end
      | 
      | if strcmp(first,last)
      |     fprintf('%s -- Copyright %s Nexteer',NxtrConf,first)
      | else
      |     fprintf('%s -- %s%s- %s Nexteer',NxtrConf,char(169),first,last)
      | end
  Product1 : Product  RndMeth=Zero
  Scope2 : Scope
      settings: SaveName=ScopeData4
  Sum2 : Sum  Inputs=|++
  Sum4 : Sum  Inputs=|+-
  Unit Delay1 : UnitDelay  SampleTime=-1  StateName=Fil2OutpPrev  StateMustResolveToSignalObject=on
      settings: AttributesFormatString=%<StateName>
  PwmPerdDither : Outport
  wires:
  Unit Delay1/1 -> Sum2/2, Sum4/2
  PWMPeriodFilt2Inp/1 -> Sum4/1
  Sum4/1 -> Product1/2
  Product1/1 -> Sum2/1
  Breakpoint Motor Velocity3/1 -> Product1/1
  Sum2/1 -> Scope2/1, PwmPerdDither/1, Unit Delay1/1

== system ES300A_SinVltgGenn/SinVltgGenn/SinVltgGennPer1 /PWMPeriodDither_U16 /RandomNumberGenerator ==
  note: Random Number range limited to 0-1
  Breakpoint Motor Velocity : Constant  Value=SINVLTGGENNSEEDMPLR_ULS_U08
  Breakpoint Motor Velocity1 : Constant  Value=SINVLTGGENNSEEDOFFS_ULS_F32
  Breakpoint Motor Velocity11 : Constant  OutDataTypeStr=single
  Breakpoint Motor Velocity2 : Constant  Value=SINVLTGGENNSEEDINI_ULS_F32
  CopyRight2 : Subsystem  Description=|  mask(Copyright Information){none=on}
      | Copyright info block.                                               
      |                                                                     
      | Place copyright information at the top of every subsystem in design.
      mask prompts: none "No parameters"
      mask help: Place copyright information at the top of every subsystem in design.
      mask Display:
      | NxtrConf = 'Nexteer Confidential';
      | 
      | sys = bdroot; %handle for the current model ("system")
      | first = get_param(sys,'Created');
      | first = first(end-3:end);  %year is last four digits
      | 
      | last = get_param(sys,'LastModifiedDate');
      | if isempty(last)
      |     last = datestr(now,'yyyy');
      | else
      |     last = last(end-3:end);
      | end
      | 
      | if strcmp(first,last)
      |     fprintf('%s -- Copyright %s Nexteer',NxtrConf,first)
      | else
      |     fprintf('%s -- %s%s- %s Nexteer',NxtrConf,char(169),first,last)
      | end
  Delay : Delay  DelayLength=1  InitialConditionSource=Input port  InitialCondition=0  StateName=RndNrPrev
      settings: AttributesFormatString=%<StateName>  InputPortMap=u0,p4
  Math Function : Math  Operator=mod  SaturateOnIntegerOverflow=on
  Product4 : Product  RndMeth=Zero
  Scope : Scope
      settings: SaveName=ScopeData6
  Sum : Sum  Inputs=|++
  RndNr : Outport  OutDataTypeStr=single
  wires:
  Product4/1 -> Sum/1
  Breakpoint Motor Velocity/1 -> Product4/2
  Breakpoint Motor Velocity1/1 -> Sum/2
  Delay/1 -> Product4/1
  Sum/1 -> Math Function/1
  Breakpoint Motor Velocity11/1 -> Math Function/2
  Math Function/1 -> Delay/1, RndNr/1, Scope/1
  Breakpoint Motor Velocity2/1 -> Delay/2

== system ES300A_SinVltgGenn/SinVltgGenn/SinVltgGennPer1 /Subsystem1/CopyRight2 ==
